simulink model "lead_compensator_with_parameter_change"  (R2023b)
settings: Solver=VariableStepAuto  StartTime=0.0  StopTime=0.05  RelTol=1e-3
settings Model: Creator=kijun  LastModifiedBy=kijun

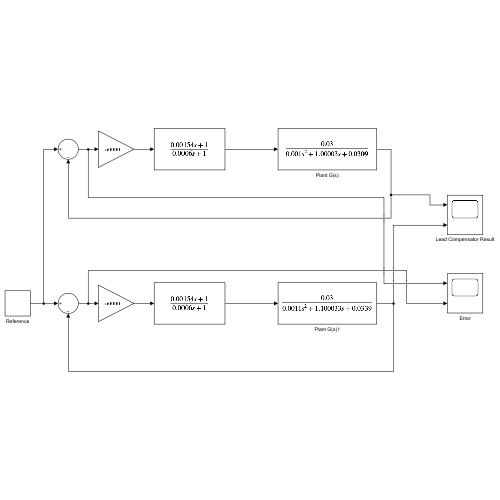
[thumbnail: Simulink's stored preview of the top-level diagram]
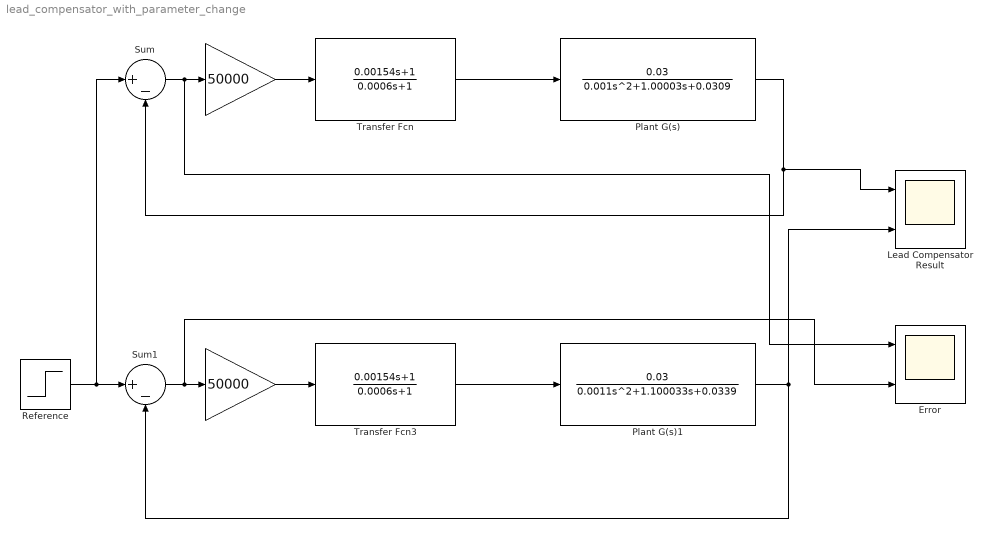
== system lead_compensator_with_parameter_change ==
  " " : Gain  Gain=50000
  "   " : Gain  Gain=50000
  Error : Scope  NumInputPorts=2
  Lead Compensator Result : Scope  NumInputPorts=2
  Plant G(s) : TransferFcn  Numerator=[0.03]  Denominator=[0.001 1.00003 0.0309]
  Plant G(s)1 : TransferFcn  Numerator=[0.03]  Denominator=[0.0011 1.100033 0.0339]
  Reference : Step  Time=0  SampleTime=0
  Sum : Sum  Inputs=|+-
  Sum1 : Sum  Inputs=|+-
  Transfer Fcn : TransferFcn  Numerator=[0.00154 1]  Denominator=[0.0006 1]
  Transfer Fcn3 : TransferFcn  Numerator=[0.00154 1]  Denominator=[0.0006 1]
  wires:
  Sum/1 -> Error/1, " "/1
  Transfer Fcn/1 -> Plant G(s)/1
  Plant G(s)/1 -> Lead Compensator Result/1, Sum/2
  " "/1 -> Transfer Fcn/1
  Reference/1 -> Sum/1, Sum1/1
  Transfer Fcn3/1 -> Plant G(s)1/1
  "   "/1 -> Transfer Fcn3/1
  Sum1/1 -> Error/2, "   "/1
  Plant G(s)1/1 -> Sum1/2, Lead Compensator Result/2
